simulink model "pidcontroller"  (R2021a)
settings: Solver=VariableStepAuto  StartTime=0.0  StopTime=10.0  RelTol=1e-3
settings Model: Creator=jameshong  LastModifiedBy=jameshong

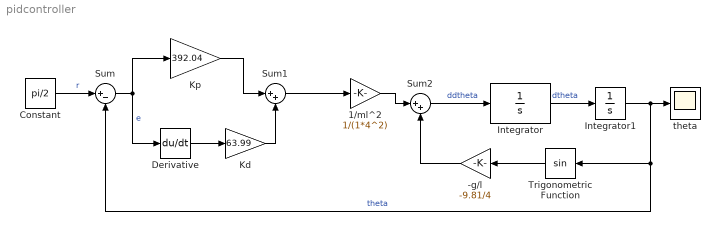
== system pidcontroller ==
  -g/l : Gain  Gain=-9.81/4
  1/ml^2 : Gain  Gain=1/(1*4^2)
  Constant : Constant  Value=pi/2
  Derivative : Derivative
  Integrator : Integrator
  Integrator1 : Integrator  InitialCondition=pi/4
  Kd : Gain  Gain=63.99
  Kp : Gain  Gain=392.04
  Sum : Sum  Inputs=|+-
  Sum1 : Sum  Inputs=|++
  Sum2 : Sum  Inputs=|++
  Trigonometric Function : Trigonometry
  theta : Scope
  wires:
  Trigonometric Function/1 -> -g/l/1
  Integrator/1 -> Integrator1/1  "dtheta"
  Integrator1/1 -> Trigonometric Function/1, Sum/2, theta/1  "theta"
  1/ml^2/1 -> Sum2/1
  -g/l/1 -> Sum2/2
  Sum2/1 -> Integrator/1  "ddtheta"
  Sum/1 -> Kp/1, Derivative/1  "e"
  Sum1/1 -> 1/ml^2/1
  Constant/1 -> Sum/1  "r"
  Derivative/1 -> Kd/1
  Kp/1 -> Sum1/1
  Kd/1 -> Sum1/2
